simulink model "chap5_6sim"  (Simulink 8.3)
settings: Solver=ode45  StartTime=0.0  StopTime=5  FixedStep=0.001  RelTol=1e-3
settings Model: Creator=ljk  LastModifiedBy=Administrator  ExtModeTrigMode=oneshot  ExtModeArmWhenConnect=off
settings DataIOCC: LimitDataPoints=off  SignalLoggingName=sigsOut
settings OptimizationCC: BooleanDataType=off  ExpressionDepthLimit=2147483647
settings DebuggingCC: SaveWithParameterizedLinksMsg=none  SignalResolutionControl=TryResolveAllWithWarning  SolverPrmCheckMsg=none  MultiTaskDSMMsg=warning  MultiTaskCondExecSysMsg=none  FcnCallInpInsideContextMsg=UseLocalSettings
settings HardwareCC: TargetUnknown=on
settings RTWCC: IncludeERTFirstTime=on

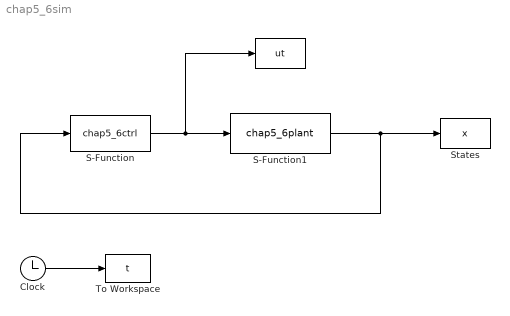
== system chap5_6sim ==
  "  " : ToWorkspace  VariableName=ut  SampleTime=-1
  Clock : Clock
  S-Function : S-Function  FunctionName=chap5_6ctrl  EnableBusSupport=off
  S-Function1 : S-Function  FunctionName=chap5_6plant  EnableBusSupport=off
  States : ToWorkspace  VariableName=x  SampleTime=-1
  To Workspace : ToWorkspace  VariableName=t  SampleTime=-1
  wires:
  S-Function/1 -> S-Function1/1, "  "/1
  S-Function1/1 -> S-Function/1, States/1
  Clock/1 -> To Workspace/1
